simulink model "Button_and_LED"  (R2023b)
settings: Solver=FixedStepAuto  StartTime=0.0  StopTime=10.0  FixedStep=1e-3  RelTol=1e-3  EnableMultiTasking=on
libraries: frdmk64flib x4
settings Model: ExtModeTrigDuration=5  Creator=bardiased  LastModifiedBy=bardiased
settings OptimizationCC: EnhancedBackFolding=on  PassReuseOutputArgsAs=Individual arguments  ZeroExternalMemoryAtStartup=off  ZeroInternalMemoryAtStartup=off  MaxStackSize=64  OptimizeBlockOrder=speed  DifferentSizesBufferReuse=on  OptimizationCustomize=off  EfficientTunableParamExpr=on
settings DebuggingCC: ParameterTunabilityLossMsg=error
settings HardwareCC: ProdBitPerPointer=32  ProdBitPerSizeT=32  ProdBitPerPtrDiffT=32  ProdLargestAtomicInteger=Long  ProdLargestAtomicFloat=Double  ProdWordSize=32  ProdHWDeviceType=ARM Compatible->ARM Cortex
settings SFSimCC: MATLABDynamicMemAlloc=off
settings RTWCC: Description=Embedded Coder  SystemTargetFile=ert.tlc  HardwareBoard=NXP FRDM-K64F  TLCOptions="-aInlineSetEventsForThisBaseRateFcn=TLC_FALSE -aSuppressMultiTaskScheduler=TLC_FALSE  -aRateBasedStepFcn=0"  TemplateMakefile=ert_default_tmf  Toolchain=GNU Tools for ARM Embedded Processors
settings CodeAppCC: ForceParamTrailComments=on  IgnoreCustomStorageClasses=off  OperatorAnnotations=on  SimulinkDataObjDesc=on  SFDataObjDesc=on  InsertBlockDesc=on
settings ERTTargetCC: ExtModeTransport=4  ExtModeMexFile=sendToCommService

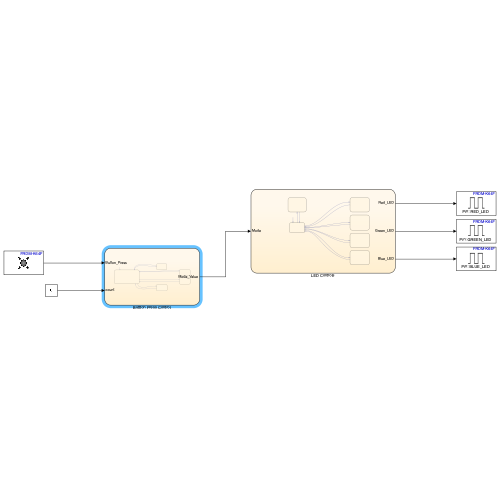
[thumbnail: Simulink's stored preview of the top-level diagram]
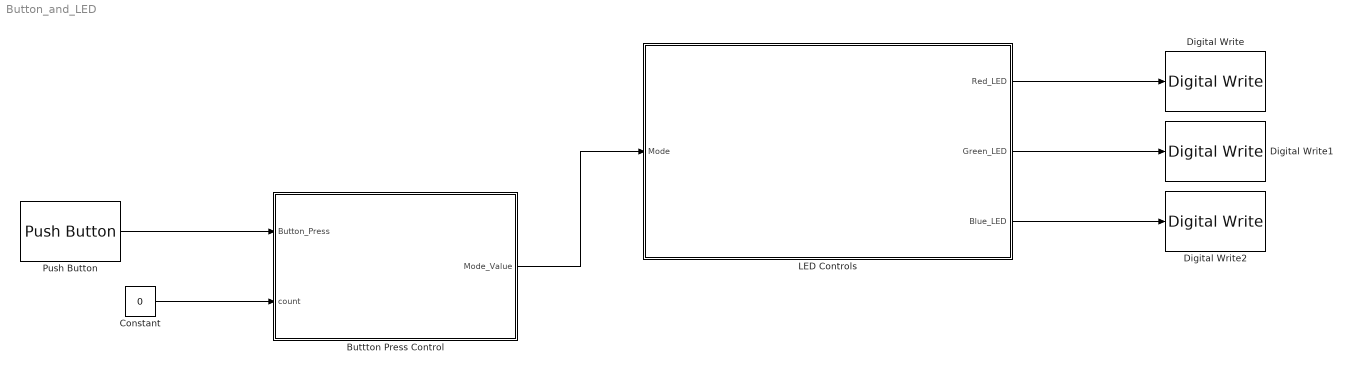
== system Button_and_LED ==
  Buttton Press Control : Stateflow chart  TreatAsAtomicUnit=on
  Constant : Constant  Value=0
  Digital Write : frdmk64flib/Digital Write  Whichpin=RED_LED
  Digital Write1 : frdmk64flib/Digital Write  Whichpin=GREEN_LED
  Digital Write2 : frdmk64flib/Digital Write  Whichpin=BLUE_LED
  LED Controls : Stateflow chart  TreatAsAtomicUnit=on
  Push Button : frdmk64flib/Push Button  Whichswitch=SW3  SampleTime1=-1
  wires:
  Push Button/1 -> Buttton Press Control/1(Button_Press)
  Constant/1 -> Buttton Press Control/2(count)
  LED Controls/1(Red_LED) -> Digital Write/1
  LED Controls/2(Green_LED) -> Digital Write1/1
  LED Controls/3(Blue_LED) -> Digital Write2/1
  Buttton Press Control/1(Mode_Value) -> LED Controls/1(Mode)

== stateflow chart Button_and_LED/LED Controls ==
  state OFF
    entry:
    Red_LED = 0
    Green_LED = 0
    Blue_LED = 0
  state AOO
    entry:
    Red_LED = 1
    Green_LED = 0
    Blue_LED = 0
  state VOO
    entry:
    Red_LED = 0
    Green_LED = 1
    Blue_LED = 0
  state Controller
  state AAI
    entry:
    Red_LED = 0
    Green_LED = 0
    Blue_LED = 1
  state VVI
    entry:
    Red_LED = 1
    Green_LED = 0
    Blue_LED = 1
  Controller -> AOO [order 2] : [Mode == 1]
  AOO -> Controller
  Controller -> OFF [order 1] : [Mode == 0]
  OFF -> Controller
  (default) -> Controller
  Controller -> VOO [order 3] : [Mode == 2]
  VOO -> Controller
  Controller -> AAI [order 4] : [Mode == 3]
  AAI -> Controller
  Controller -> VVI [order 5] : [Mode == 4]
  VVI -> Controller
  data: Mode input; Red_LED output; Green_LED output; Blue_LED output

== stateflow chart Button_and_LED/Buttton Press Control ==
  state AOO
    entry:
    Mode_Value = 1
  state VOO
    entry:
    Mode_Value = 2
  state Controller
    entry:
    counter = 1 + mod(counter,4) %mod  4
  state AAI
    entry:
    Mode_Value = 3
  state VVI
    entry:
    Mode_Value = 4
  AOO -> Controller : [Button_Press == 0]
  Controller -> AOO [order 1] : [Button_Press == 1 && counter == 1]
  (default) -> Controller
  Controller -> VOO [order 2] : [Button_Press  == 1 && counter == 2]
  VOO -> Controller : [Button_Press  == 0]
  Controller -> AAI [order 3] : [Button_Press  == 1 && counter == 3]
  AAI -> Controller : [Button_Press  == 0]
  VVI -> Controller : [Button_Press  == 0]
  Controller -> VVI [order 4] : [Button_Press  == 1 && counter == 4]
  data: Mode_Value output; Button_Press input; count input; counter local =0
